simulink model "SimulacaoMaquinaCCTorqueVariavel"  (R2022a)
settings: Solver=VariableStepAuto  StartTime=0.0  StopTime=10  MaxStep=1e-4  RelTol=1e-3
libraries: spsControlledVoltageSourceLib x1, spsDCVoltageSourceLib x1, spsVoltageMeasurementLib x1, spsDCMachineLib x1, simulink x1, spspowerguiLib x1
settings Model: Creator=marcone.faria  LastModifiedBy=marcone.faria

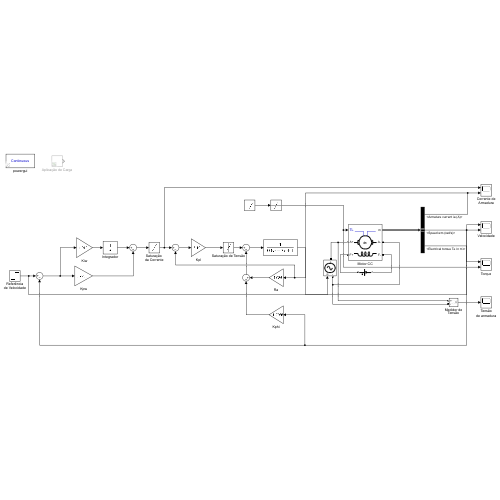
[thumbnail: Simulink's stored preview of the top-level diagram]
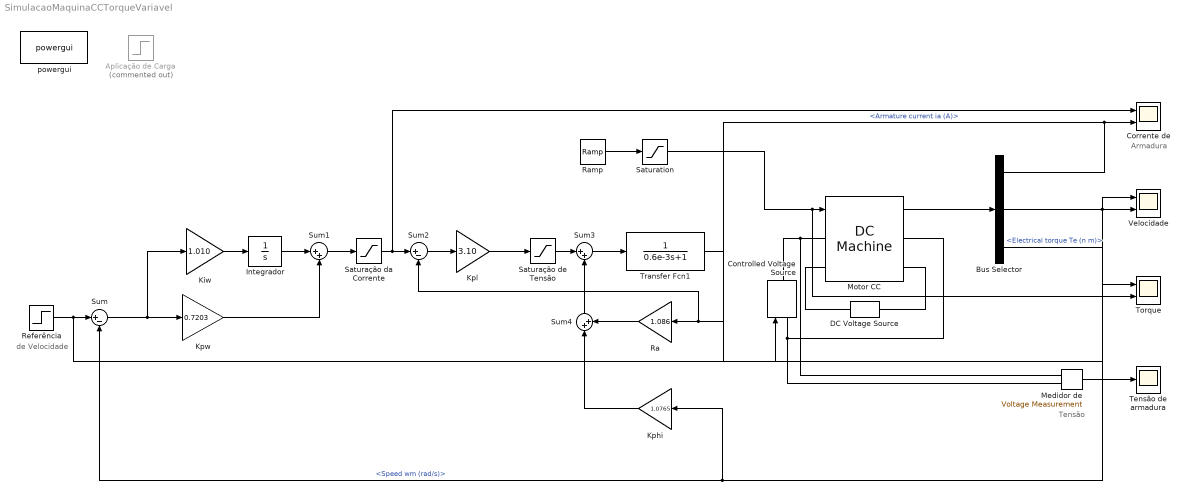
== system SimulacaoMaquinaCCTorqueVariavel ==
  note: Tensão
  note: Armadura
  note: de Velocidade
  Aplicação de Carga : Step  Commented=on  After=20  SampleTime=0
  Bus Selector : BusSelector  OutputSignals=Armature current ia (A),Speed wm (rad/s),Electrical torque Te (n m)
  Controlled Voltage Source : spsControlledVoltageSourceLib/Controlled Voltage Source  Initialize=on  Source_Type=AC  Amplitude=0  Phase=0  Frequency=0  Measurements=None
  Corrente de : Scope  NumInputPorts=2
  DC Voltage Source : spsDCVoltageSourceLib/DC Voltage Source  Amplitude=300  Measurements=None
  Integrador : TransferFcn  Denominator=[1 0]
  Kiw : Gain  Gain=1.010
  Kphi : Gain  Gain=1.0765
  Kpl : Gain  Gain=3.10
  Kpw : Gain  Gain=0.7203
  Medidor de : spsVoltageMeasurementLib/Voltage Measurement  PhasorSimulation=off  OutputType=Complex  PSBequivalent=0
  Motor CC : spsDCMachineLib/DC Machine  PresetModel=04: 10HP 240V 1750RPM Field:300V  MechanicalLoad=Torque TL  FieldType=Wound  ShowDetailedParameters=on  MeasurementBus=off  RLa=[1.086 0.01216]  RLf=[180 71.47]  Laf=0.6458  MachineConstant=Torque constant (N.m/A)  Ke=1.8  Kt=1.8  J=0.04251  Bm=0.003406  Tf=1.046  w0=1  Ifinit=1.66666666666667  TsPowergui=0  TsBlock=-1
  Ra : Gain  Gain=1.086
  Ramp : simulink/Sources/Ramp  slope=1000  start=3  InitialOutput=0
  Referência : Step  After=92  SampleTime=0
  Saturation : Saturate  UpperLimit=40  LowerLimit=20
  Saturação da Corrente : Saturate  UpperLimit=72  LowerLimit=-72
  Saturação de Tensão : Saturate  UpperLimit=360  LowerLimit=-360
  Sum : Sum  Inputs=|+-
  Sum1 : Sum  Inputs=|++
  Sum2 : Sum  Inputs=|+-
  Sum3 : Sum  Inputs=|++
  Sum4 : Sum  Inputs=|++
  Tensão de armadura : Scope
  Torque : Scope  NumInputPorts=2
  Transfer Fcn1 : TransferFcn  Denominator=[0.6e-3 1]
  Velocidade : Scope  NumInputPorts=2
  powergui : spspowerguiLib/powergui  Priority=1  SimulationMode=Continuous  SampleTime=50e-6  frequency=60  Iterations=50  frequencyindice=0  Pbase=100e6  ErrMax=1e-4  UnitsV=kV  UnitsW=MW  buscounter=0  FunctionMessages=off  echomessages=off  EnableUseOfTLC=off  CurrentSourceSwitches=off  DisableSnubberDevices=off  DisableRonSwitches=off  DisableVfSwitches=off  DisplayEquations=off  AutomaticDiscreteSolvers=off  SolverType=Tustin/Backward Euler (TBE)  Interpol=off  ExternalGateDelay=off  methode=off  Ts=100  x0status=blocks  SPID=on  SwTol=0  HookPort=off  NonlinearTolerance=1e-4  nMaxIteration=100  ContinueOnMaxIteration=off  RestoreLinks=warning  ResistiveCurrentMeasurement=off  Frange=[0:2:500]  Ylog=off  Xlog=on  ShowGrid=off  save=off  variable=ZData  structure=0  ZoomFFT=off  StartTime=0.0  cycles=1  DisplayStyle=1  fundamental=60  FreqAxis=off  MaxFrequency=1000  frequencyindicesteady=1  RmsSteady=1  display=off
  wires:
  Transfer Fcn1/1 -> Controlled Voltage Source/1
  Referência/1 -> Velocidade/1, Sum/1
  Sum/1 -> Kiw/1, Kpw/1
  Kiw/1 -> Integrador/1
  Integrador/1 -> Sum1/1
  Kpw/1 -> Sum1/2
  Sum1/1 -> Saturação da Corrente/1
  Saturação da Corrente/1 -> Corrente de/1, Sum2/1
  Sum2/1 -> Kpl/1
  Kpl/1 -> Saturação de Tensão/1
  Saturação de Tensão/1 -> Sum3/1
  Sum3/1 -> Transfer Fcn1/1
  Sum4/1 -> Sum3/2
  Ra/1 -> Sum4/2
  Kphi/1 -> Sum4/1
  Saturation/1 -> Motor CC/1, Torque/2
  Medidor de/1 -> Tensão de armadura/1
  Motor CC/1 -> Bus Selector/1
  Bus Selector/1 -> Sum2/2, Ra/1, Corrente de/2  "<Armature current ia (A)>"
  Bus Selector/2 -> Velocidade/2, Kphi/1, Sum/2  "<Speed wm (rad/s)>"
  Bus Selector/3 -> Torque/1  "<Electrical torque Te (n m)>"
  Ramp/1 -> Saturation/1
  connections:
  Motor CC/RConn2 -- DC Voltage Source/LConn1
  Motor CC/LConn2 -- DC Voltage Source/RConn1
  Controlled Voltage Source/RConn1 -- Medidor de/LConn1 -- Motor CC/LConn1
  Controlled Voltage Source/LConn1 -- Medidor de/LConn2 -- Motor CC/RConn1
